simulink model "furuta_model"  (R2020a)
settings: Solver=VariableStepAuto  StartTime=0.0  StopTime=10.0  RelTol=1e-6
undefined symbols (not defined in the file): g, J, l_b, l_p, M, m_b, m_p, x0
settings Model: Creator=angelo  LastModifiedBy=angelo
settings ModelReferenceCC: ModelReferenceNumInstancesAllowed=Single

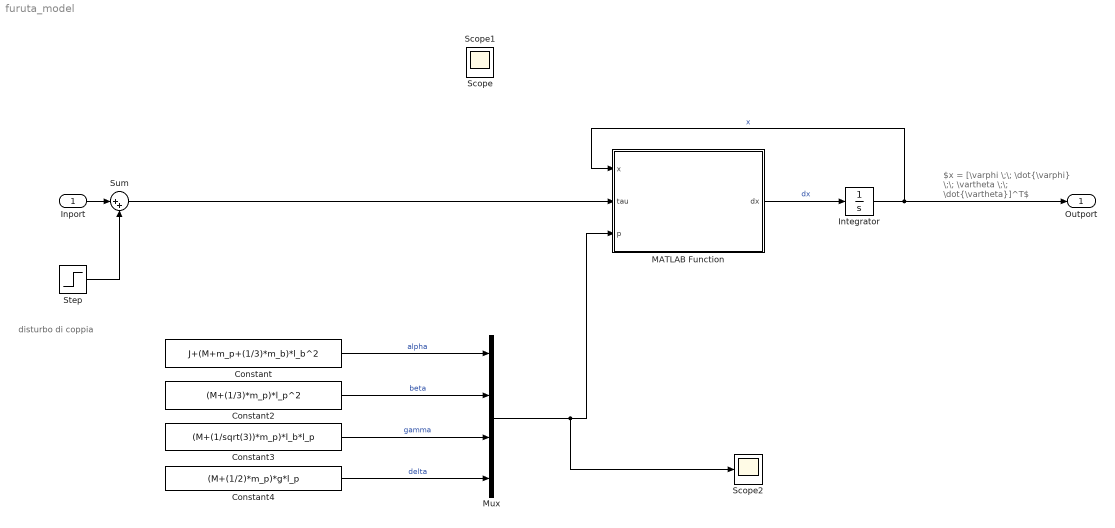
== system furuta_model ==
  note: disturbo di coppia
  note: $x = [\varphi \;\; \dot{\varphi} \;\; \vartheta \;\; \dot{\vartheta}]^T$
  Inport : Inport
  Constant : Constant  Value=J+(M+m_p+(1/3)*m_b)*l_b^2
  Constant2 : Constant  Value=(M+(1/3)*m_p)*l_p^2
  Constant3 : Constant  Value=(M+(1/sqrt(3))*m_p)*l_b*l_p
  Constant4 : Constant  Value=(M+(1/2)*m_p)*g*l_p
  Integrator : Integrator  InitialCondition=x0
  MATLAB Function : MATLAB Function  TreatAsAtomicUnit=on
  Mux : Mux
  Scope2 : Scope
  Step : Step  Time=0.1  Before=1  After=0  SampleTime=0
  Sum : Sum  Inputs=|++
  Outport : Outport
  Scope : Scope
  Scope1 : Scope
  wires:
  MATLAB Function/1(dx) -> Integrator/1  "dx"
  Integrator/1 -> Outport/1, MATLAB Function/1(x)  "x"
  Inport/1 -> Sum/1
  Step/1 -> Sum/2
  Sum/1 -> MATLAB Function/2(tau)
  Mux/1 -> Scope2/1, MATLAB Function/3(p)
  Constant/1 -> Mux/1  "alpha"
  Constant2/1 -> Mux/2  "beta"
  Constant3/1 -> Mux/3  "gamma"
  Constant4/1 -> Mux/4  "delta"

== matlab function furuta_model/MATLAB Function ==
  data: x input; tau input; dx output; p input
function dx = furuta(x, tau, p)

m_p = 0.3;  %pendulum mass [kg]
l_p = 0.205;  %pendulum length [m]
m_b = 1;  %brace mass [kg]
l_b = 0.3;  %brace length [m]
M = 1;  %puntiform mass [kg]
J = 0.1531;  %moment of inertia [kg*m^2]
g = 9.81;  %gravity [m*s^-2]

k = 2.7;  %torque drive constant [Nm/V] 
k_i = 2.667;  %drive transconductance constant [A/V]
k_g = 15;  %trasmission ratio
k_t = 0.1;  %torque motor constant [Nm/A]

b_phi = 0.337;  %viscous friction of brace [Nm s/rad]
b_theta = 0.035;  %viscous friction of pendulum [Nm s/rad]

% inizialitation
dx = zeros(4, 1);

% parameters
alpha = p(1);
beta = p(2);
gamma = p(3);
delta = p(4);

% state
phi = x(1);
dphi = x(2);
theta = x(3);  
dtheta = x(4);

% input
tau_phi = tau;
%tau_phi = tau(1);
%tau_theta = tau(2);

% common term for ddphi and ddtheta
t0 = 1/(beta*(alpha + beta*(sin(theta)^2))-gamma^2*(cos(theta)^2));

% terms of ddphi
t1 = beta*gamma*sin(theta)*(dtheta^2);
t2 = gamma*delta*cos(theta)*sin(theta);
t3 = (2*(beta^2)*cos(theta)*sin(theta))*dphi*dtheta;
t4 = gamma*b_theta*cos(theta)*dtheta;
t5 = (beta*gamma*(cos(theta)^2)*sin(theta))*(dphi^2);
t6 = beta*(tau_phi - b_phi*dphi);

% ddphi
ddphi = t0*(t1-t2-t3+t4+t5+t6);

% terms of ddtheta
t00 = (alpha + beta*(sin(theta)^2));
t1 = t00*delta*sin(theta);
t2 = t00*(beta*cos(theta)*sin(theta)*(dphi^2));
t3 = 2*beta*gamma*(cos(theta)^2)*sin(theta)*dphi*dtheta;
t4 = (gamma^2)*sin(theta)*cos(theta)*(dtheta^2);
t5 = t00*b_theta*dtheta;
t6 = gamma*cos(theta)*b_phi*dphi;
t7 = gamma*cos(theta)*tau_phi;

% ddtheta
ddtheta = t0*(t1 +t2 +t3 - t4 - t5 + t6 - t7);

% output
dx(1) = dphi;
dx(2) = ddphi;
dx(3) = dtheta;
dx(4) = ddtheta;
end
